simulink model "eval_double"  (R2014b)
settings: Solver=ode3  SolverMode=SingleTasking  StartTime=0.0  StopTime=Tsim  FixedStep=Ts  RelTol=1e-3
InitFcn:
  | configDoubleIntegrator
settings Model: CovMetricSettings=dwe  CovHtmlReporting=off  covSaveCumulativeToWorkspaceVar=off  CovSaveSingleToWorkspaceVar=off  CovExternalEMLEnable=on  CovSFcnEnable=on  Creator=mnade  LastModifiedBy=nina
settings DataIOCC: LimitDataPoints=off  SaveFormat=StructureWithTime
settings DebuggingCC: SolverPrmCheckMsg=none  FrameProcessingCompatibilityMsg=error  SFUnexpectedBacktrackingDiag=error  SFNoUnconditionalDefaultTransitionDiag=error
settings HardwareCC: ProdBitPerPointer=64  ProdLargestAtomicFloat=Float  ProdIntDivRoundTo=Zero  ProdEndianess=LittleEndian  ProdHWDeviceType=Specified
settings ModelReferenceCC: PropagateSignalLabelsOutOfModel=on
settings GRTTargetCC: TargetLangStandard=C99 (ISO)  GeneratePreprocessorConditionals=Use local settings

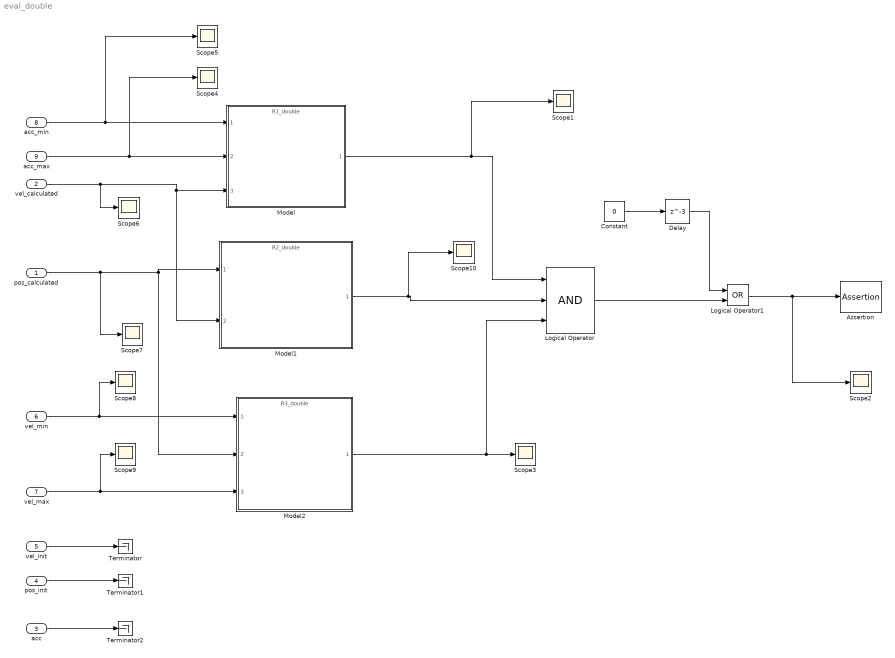
== system eval_double ==
  pos_calculated : Inport
  vel_calculated : Inport  Port=2
  acc : Inport  Port=3
  pos_init : Inport  Port=4
  vel_init : Inport  Port=5
  vel_min : Inport  Port=6
  vel_max : Inport  Port=7
  acc_min : Inport  Port=8
  acc_max : Inport  Port=9
  Assertion : Assertion  StopWhenAssertionFail=off
  Constant : Constant  Value=0
  Delay : Delay  DelayLength=3  InitialCondition=1
  Logical Operator : Logic  Inputs=3  AllPortsSameDT=off  OutDataTypeStr=boolean
  Logical Operator1 : Logic  Operator=OR  AllPortsSameDT=off  OutDataTypeStr=boolean
  Model : ModelReference  ModelNameDialog=R1_double.slx  SimulationMode=Normal  ModelReferenceVersion=1.14  CopyOfModelName=R1_double.slx  DefaultDataLogging=on
  Model1 : ModelReference  ModelNameDialog=R2_double.slx  SimulationMode=Normal  ModelReferenceVersion=1.18  CopyOfModelName=R2_double.slx  DefaultDataLogging=on
  Model2 : ModelReference  ModelNameDialog=R3_double.slx  SimulationMode=Normal  ModelReferenceVersion=1.19  CopyOfModelName=R3_double.slx  DefaultDataLogging=on
  Scope{1..10} (10 alike) : Scope
      Scope2 settings: SaveName=ScopeData2
      Scope3 settings: SaveName=ScopeData3
      Scope4 settings: SaveName=ScopeData4
      Scope5 settings: SaveName=ScopeData5
      Scope6 settings: SaveName=ScopeData6
      Scope7 settings: SaveName=ScopeData7
      Scope8 settings: SaveName=ScopeData8
      Scope9 settings: SaveName=ScopeData9
  Terminator : Terminator
  Terminator1 : Terminator
  Terminator2 : Terminator
  wires:
  acc_min/1 -> Scope5/1, Model/1
  acc_max/1 -> Scope4/1, Model/2
  vel_calculated/1 -> Scope6/1, Model1/2, Model/3
  Model/1 -> Scope1/1, Logical Operator/1
  Model1/1 -> Scope10/1, Logical Operator/2
  pos_calculated/1 -> Scope7/1, Model2/2, Model1/1
  vel_min/1 -> Scope8/1, Model2/1
  Model2/1 -> Scope3/1, Logical Operator/3
  vel_max/1 -> Scope9/1, Model2/3
  pos_init/1 -> Terminator1/1
  vel_init/1 -> Terminator/1
  acc/1 -> Terminator2/1
  Logical Operator1/1 -> Assertion/1, Scope2/1
  Logical Operator/1 -> Logical Operator1/2
  Constant/1 -> Delay/1
  Delay/1 -> Logical Operator1/1
